simulink model "DSimulator_robot"  (Simulink 8.1)
settings: Solver=ode4  StartTime=0.0  StopTime=30.0  FixedStep=0.01  RelTol=1e-3
undefined symbols (not defined in the file or in its folder): Correct_robot, Dinamic_robot
libraries: roblocks x1
settings Model: Creator=E. Dean  LastModifiedBy=root
settings DebuggingCC: StrictBusMsg=Warning

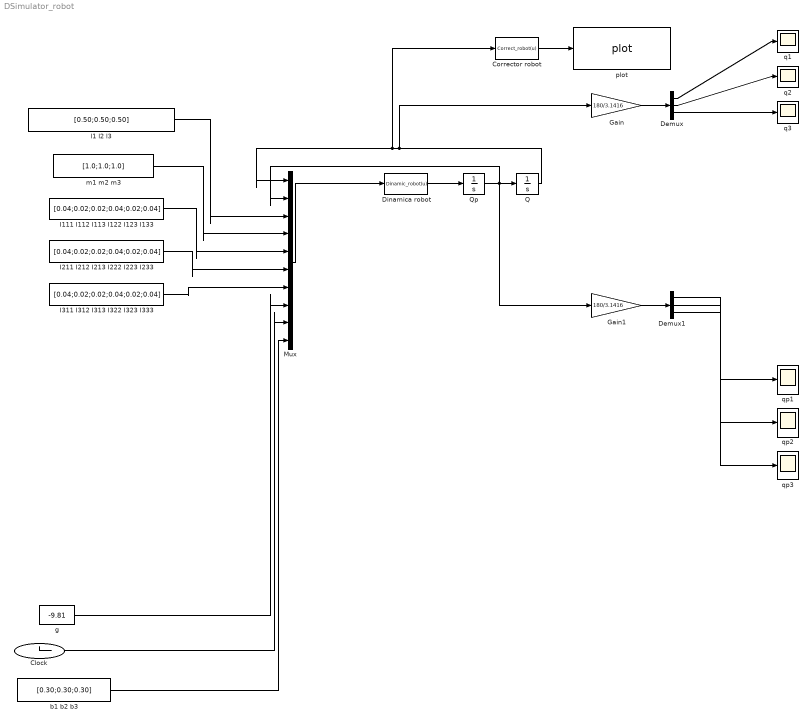
== system DSimulator_robot ==
  Clock : Clock
      settings: Decimation=100
  Corrector robot : MATLABFcn  MATLABFcn=Correct_robot(u)  OutputDimensions=3
  Demux : Demux  Outputs=3
  Demux1 : Demux  Outputs=3
  Dinamica robot : MATLABFcn  MATLABFcn=Dinamic_robot(u)  OutputDimensions=3
  Gain : Gain  Gain=180/3.1416
  Gain1 : Gain  Gain=180/3.1416
  I111 I112 I113 I122 I123 I133 : Constant  Value=[0.04;0.02;0.02;0.04;0.02;0.04]
  I211 I212 I213 I222 I223 I233 : Constant  Value=[0.04;0.02;0.02;0.04;0.02;0.04]
  I311 I312 I313 I322 I323 I333 : Constant  Value=[0.04;0.02;0.02;0.04;0.02;0.04]
  Mux : Mux  Inputs=10
  Q : Integrator  InitialCondition=[0;0;0]
  Qp : Integrator  InitialCondition=[0;0;0]
  "b1 b2 b3 " : Constant  Value=[0.30;0.30;0.30]
  g : Constant  Value=-9.81
  "l1 l2 l3 " : Constant  Value=[0.50;0.50;0.50]
  "m1 m2 m3 " : Constant  Value=[1.0;1.0;1.0]
  plot : roblocks/plot  robot=Robot_robotF
  q1 : Scope
      settings: TimeRange=10  YMin=0  YMax=55
  q2 : Scope
      settings: TimeRange=10  YMax=55
  q3 : Scope
      settings: TimeRange=10  YMin=0  YMax=40
  qp1 : Scope
  qp2 : Scope
  qp3 : Scope
  wires:
  Qp/1 -> Q/1, Gain1/1, Mux/2
  Dinamica robot/1 -> Qp/1
  Mux/1 -> Dinamica robot/1
  Q/1 -> Gain/1, Mux/1, Corrector robot/1
  Gain/1 -> Demux/1
  Demux/1 -> q1/1
  Demux/2 -> q2/1
  Demux/3 -> q3/1
  Gain1/1 -> Demux1/1
  Demux1/1 -> qp1/1
  Demux1/2 -> qp2/1
  Demux1/3 -> qp3/1
  "l1 l2 l3 "/1 -> Mux/3
  "m1 m2 m3 "/1 -> Mux/4
  I111 I112 I113 I122 I123 I133/1 -> Mux/5
  I211 I212 I213 I222 I223 I233/1 -> Mux/6
  I311 I312 I313 I322 I323 I333/1 -> Mux/7
  g/1 -> Mux/8
  Clock/1 -> Mux/9
  "b1 b2 b3 "/1 -> Mux/10
  Corrector robot/1 -> plot/1
